simulink model "P_HIL_Virtual_Env"  (R2019b)
settings: Solver=VariableStepAuto  StartTime=0.0  StopTime=0.5  MaxStep=1e-6  RelTol=1e-3
undefined symbols (not defined in the file): Apd, Apd_i_dhs, Apd_u_dhs, C_dhs, f_sw, f_sw_dhs, In, L, L_dhs, L_drom, T_sw_dhs, Tid, Tid_i_dhs, Tid_u_dhs, U_DC
libraries: coordinate_transformations x19, simulink x6, PE_components x2
settings Model: SimulationMode=accelerator  Creator=kissd  LastModifiedBy=kissd

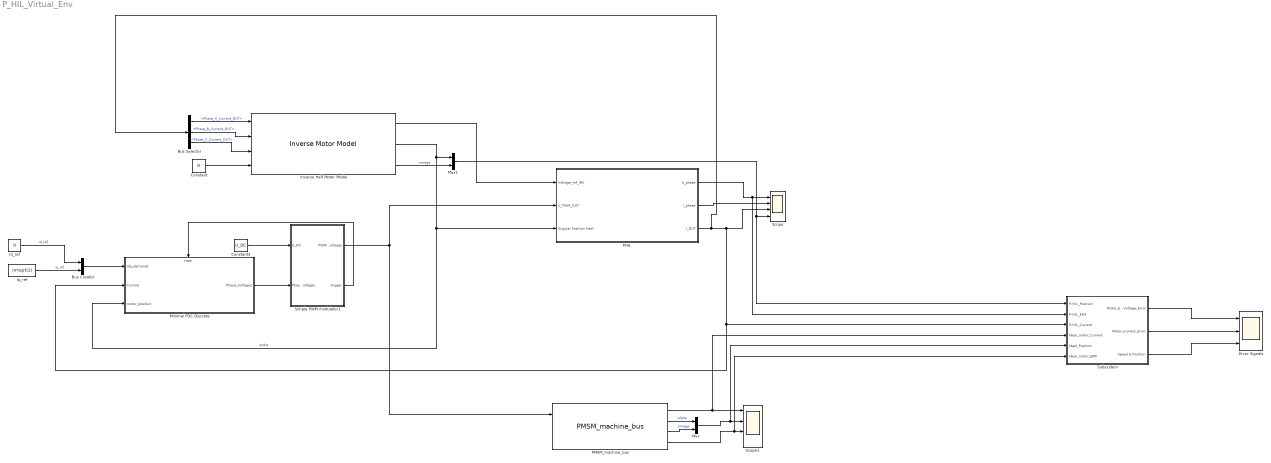
== system P_HIL_Virtual_Env ==
  Bus Creator : BusCreator  Inputs=2
  Bus Selector : BusSelector  OutputSignals=Phase_A_Current_DUT,Phase_B_Current_DUT,Phase_C_Current_DUT
  Constant : Constant  Value=0
  Constant3 : Constant  Value=U_DC
  Error Signals : Scope  NumInputPorts=3
  Inverse Half Motor Model : PE_components/Inverse Motor Model  SystemSampleTime=-1  Latency=0  AutoFrameSizeCalculation=off
  Minimal FOC Discrete : Subsystem  AncestorBlock=controllers/Minimal FOC Discrete
  Mux : Mux  Inputs=2
  Mux1 : Mux  Inputs=2
  PHIL : Subsystem
  PMSM_machine_bus : PE_components/PMSM_machine_bus  SystemSampleTime=-1  Latency=0  AutoFrameSizeCalculation=off
      link override Gain: Gain=1/Ld
      link override Gain3: Gain=1/Lq
      link override Gain8: Gain=Lq
  Scope : Scope  NumInputPorts=4
  Scope1 : Scope  NumInputPorts=4
  Simple PWM modulator1 : Subsystem  AncestorBlock=controllers/Simple PWM modulator
  Subsystem : Subsystem
  id_ref : Constant  Value=0
  iq_ref : Constant  Value=In*sqrt(2)
  wires:
  Constant3/1 -> Simple PWM modulator1/1(U_DC)
  id_ref/1 -> Bus Creator/1  "id_ref"
  iq_ref/1 -> Bus Creator/2  "iq_ref"
  Minimal FOC Discrete/1(Phase_Voltages) -> Simple PWM modulator1/2(Phase_Voltages)
  Simple PWM modulator1/2(trigger) -> Minimal FOC Discrete/Trigger
  Bus Creator/1 -> Minimal FOC Discrete/1(Idq_demands)
  Simple PWM modulator1/1(PWM_Voltages) -> PHIL/2("U_PWM_DUT "), PMSM_machine_bus/1
  PHIL/1(U_phase) -> Subsystem/2(P-HIL_EMF), Scope/1
  PHIL/2(I_phase) -> Scope/2
  PHIL/3(I_DUT) -> Bus Selector/1, Minimal FOC Discrete/2(Current), Subsystem/3(P-HIL_Current), Scope/3
  Inverse Half Motor Model/1 -> PHIL/1(Voltage_ref_INV)
  Bus Selector/1 -> Inverse Half Motor Model/1  "<Phase_A_Current_DUT>"
  Bus Selector/2 -> Inverse Half Motor Model/2  "<Phase_B_Current_DUT>"
  Bus Selector/3 -> Inverse Half Motor Model/3  "<Phase_C_Current_DUT>"
  Inverse Half Motor Model/3 -> Mux1/2  "omega"
  PMSM_machine_bus/1 -> Subsystem/4(Ideal_motor_Current), Scope1/1
  PMSM_machine_bus/4 -> Subsystem/6(Ideal_motor_EMF), Scope1/3
  PMSM_machine_bus/2 -> Mux/1  "alpha"
  PMSM_machine_bus/3 -> Mux/2  "omega"
  Mux/1 -> Subsystem/5(Ideal_Position), Scope1/2
  Inverse Half Motor Model/2 -> Mux1/1, Minimal FOC Discrete/3(motor_position), PHIL/3(Angular Position (rad))  "alpha"
  Mux1/1 -> Subsystem/1(P-HIL_Position), Scope/4
  Constant/1 -> Inverse Half Motor Model/4
  Subsystem/1(Motor_EMF_Voltage_Error) -> Error Signals/1
  Subsystem/2(Motor_Current_Error) -> Error Signals/2
  Subsystem/3(Speed & Position) -> Error Signals/3

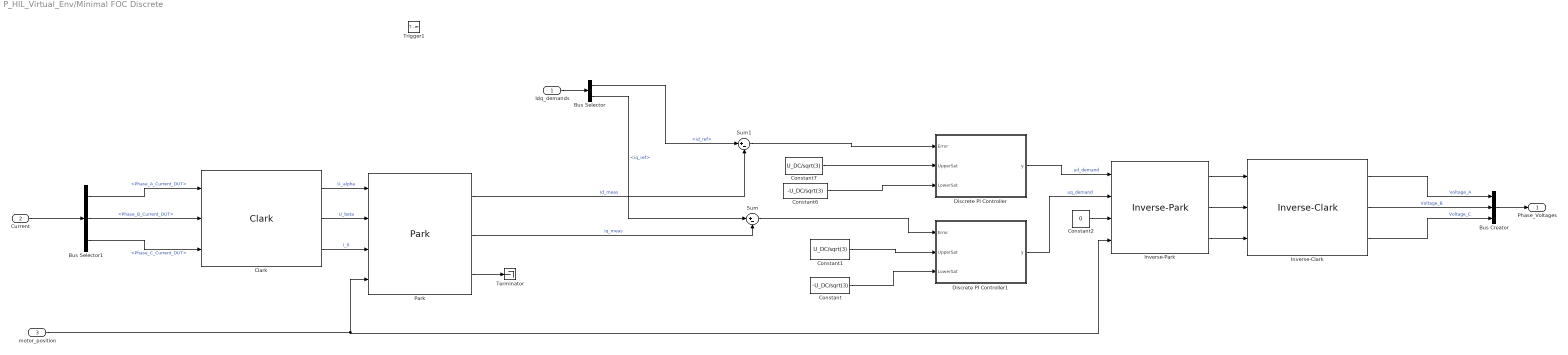
== system P_HIL_Virtual_Env/Minimal FOC Discrete ==
  Idq_demands : Inport
  Current : Inport  Port=2
  motor_position : Inport  Port=3
  Trigger1 : TriggerPort  TriggerType=either  VariantControl=Variant  PortDimensions=1
  Bus Creator : BusCreator  Inputs=3
  Bus Selector : BusSelector  OutputSignals=id_ref,iq_ref
  Bus Selector1 : BusSelector  OutputSignals=Phase_A_Current_DUT,Phase_B_Current_DUT,Phase_C_Current_DUT
  Clark : coordinate_transformations/Clark  SystemSampleTime=-1  Latency=0  AutoFrameSizeCalculation=off
  Constant : Constant  Value=-U_DC/sqrt(3)
  Constant1 : Constant  Value=U_DC/sqrt(3)
  Constant2 : Constant  Value=0
  Constant6 : Constant  Value=-U_DC/sqrt(3)
  Constant7 : Constant  Value=U_DC/sqrt(3)
  Discrete PI Controller : Subsystem  AncestorBlock=controllers/Discrete PI Controller  mask(Continous PI Controller){Apd=Apd, Tid=Tid, fs=f_sw}
      mask prompts: Apd "Proprotional Gain"; Tid "Integration Time"; fs "fsw"
      mask help: Continous PI Controller description.
  Discrete PI Controller1 : Subsystem  AncestorBlock=controllers/Discrete PI Controller  mask(Continous PI Controller){Apd=Apd, Tid=Tid, fs=f_sw}
      mask prompts: Apd "Proprotional Gain"; Tid "Integration Time"; fs "fsw"
      mask help: Continous PI Controller description.
  Inverse-Clark : coordinate_transformations/Inverse-Clark  SystemSampleTime=-1  Latency=0  AutoFrameSizeCalculation=off
  Inverse-Park : coordinate_transformations/Inverse-Park  SystemSampleTime=-1  Latency=0  AutoFrameSizeCalculation=off
  Park : coordinate_transformations/Park  SystemSampleTime=-1  Latency=0  AutoFrameSizeCalculation=off
  Sum : Sum  Inputs=|+-
  Sum1 : Sum  Inputs=|+-
  Terminator : Terminator
  Phase_Voltages : Outport
  wires:
  Discrete PI Controller1/1(y) -> Inverse-Park/2  "uq_demand"
  Inverse-Park/2 -> Inverse-Clark/2
  Inverse-Park/3 -> Inverse-Clark/3
  Park/2 -> Sum/2  "Iq_meas"
  Constant7/1 -> Discrete PI Controller/2(UpperSat)
  Clark/1 -> Park/1  "U_alpha"
  Inverse-Clark/3 -> Bus Creator/3  "Voltage_C"
  Constant1/1 -> Discrete PI Controller1/2(UpperSat)
  Sum/1 -> Discrete PI Controller1/1(Error)
  Inverse-Park/1 -> Inverse-Clark/1
  Constant6/1 -> Discrete PI Controller/3(LowerSat)
  motor_position/1 -> Park/4, Inverse-Park/4
  Park/1 -> Sum1/2  "Id_meas"
  Discrete PI Controller/1(y) -> Inverse-Park/1  "ud_demand"
  Constant/1 -> Discrete PI Controller1/3(LowerSat)
  Sum1/1 -> Discrete PI Controller/1(Error)
  Clark/2 -> Park/2  "U_beta"
  Bus Selector/2 -> Sum/1  "<iq_ref>"
  Clark/3 -> Park/3  "I_0"
  Park/3 -> Terminator/1
  Inverse-Clark/2 -> Bus Creator/2  "Voltage_B"
  Bus Selector/1 -> Sum1/1  "<id_ref>"
  Inverse-Clark/1 -> Bus Creator/1  "Voltage_A"
  Current/1 -> Bus Selector1/1
  Constant2/1 -> Inverse-Park/3
  Idq_demands/1 -> Bus Selector/1
  Bus Creator/1 -> Phase_Voltages/1
  Bus Selector1/2 -> Clark/2  "<Phase_B_Current_DUT>"
  Bus Selector1/1 -> Clark/1  "<Phase_A_Current_DUT>"
  Bus Selector1/3 -> Clark/3  "<Phase_C_Current_DUT>"

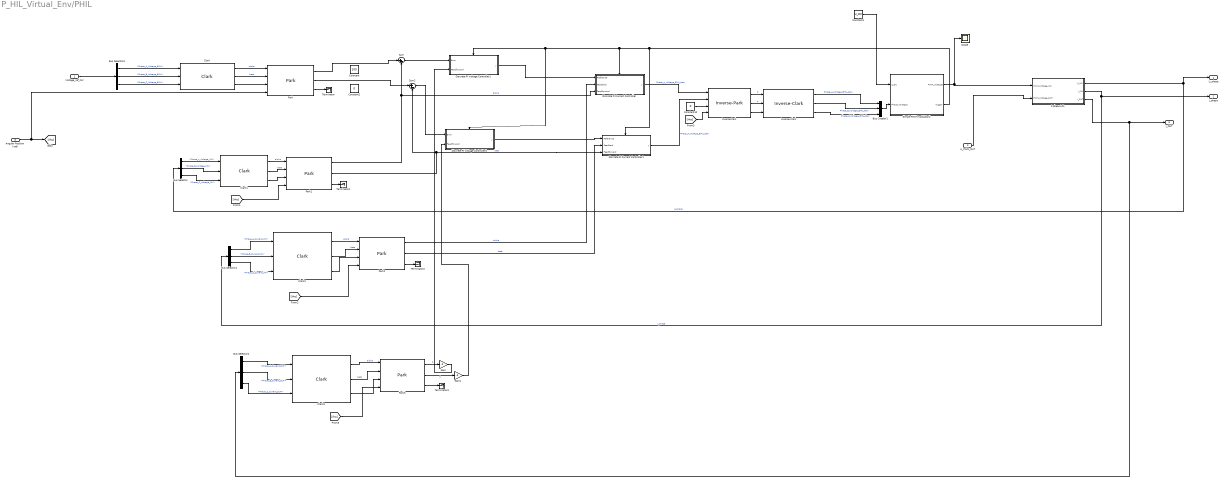
== system P_HIL_Virtual_Env/PHIL ==
  Voltage_ref_INV : Inport
  "U_PWM_DUT " : Inport  Port=2
  Angular Position (rad) : Inport  Port=3
  3 phase LCL : Subsystem
  Bus Creator1 : BusCreator  Inputs=3
  Bus Selector : BusSelector  OutputSignals=Phase_A_Voltage_INV,Phase_B_Voltage_INV,Phase_C_Voltage_INV
  Bus Selector1 : BusSelector  OutputSignals=Phase_A_Current_INV,Phase_B_Current_INV,Phase_C_Current_INV
  Bus Selector2 : BusSelector  OutputSignals=Phase_A_Current_DUT,Phase_B_Current_DUT,Phase_C_Current_DUT
  Bus Selector3 : BusSelector  OutputSignals=Phase_A_Voltage_EMU,Phase_B_Voltage_EMU,Phase_C_Voltage_EMU
  Clark{,1..3} (4 alike) : coordinate_transformations/Clark  SystemSampleTime=-1  Latency=0  AutoFrameSizeCalculation=off
  Constant : Constant  Value=100
  Constant1 : Constant  Value=U_DC
  Constant10 : Constant  Value=0
  Constant2 : Constant  Value=0
  Discrete PI Current Controller : Subsystem  AncestorBlock=controllers/Discrete PI Controller  mask(Continous PI Controller){Apd=Apd_i_dhs, Tid=Tid_i_dhs, fs=f_sw_dhs, UpperSat=U_DC, LowerSat=-U_DC}
      mask prompts: Apd "Proprotional Gain"; Tid "Integration Time"; fs "fsw"; UpperSat "Max. Saturation"; LowerSat "Min. Saturation"
      mask help: Continous PI Controller description.
  Discrete PI Current Controller1 : Subsystem  AncestorBlock=controllers/Discrete PI Controller  mask(Continous PI Controller){Apd=Apd_i_dhs, Tid=Tid_i_dhs, fs=f_sw_dhs, UpperSat=U_DC, LowerSat=-U_DC}
      mask prompts: Apd "Proprotional Gain"; Tid "Integration Time"; fs "fsw"; UpperSat "Max. Saturation"; LowerSat "Min. Saturation"
      mask help: Continous PI Controller description.
  Discrete PI Voltage Controller1 : Subsystem  AncestorBlock=controllers/Discrete PI Controller  mask(Continous PI Controller){Apd=Apd_u_dhs, Tid=Tid_u_dhs, fs=f_sw_dhs, UpperSat=300, LowerSat=-300}
      mask prompts: Apd "Proprotional Gain"; Tid "Integration Time"; fs "fsw"; UpperSat "Max. Saturation"; LowerSat "Min. Saturation"
      mask help: Continous PI Controller description.
  Discrete PI Voltage Controller3 : Subsystem  AncestorBlock=controllers/Discrete PI Controller  mask(Continous PI Controller){Apd=Apd_u_dhs, Tid=Tid_u_dhs, fs=f_sw_dhs, UpperSat=300, LowerSat=-300}
      mask prompts: Apd "Proprotional Gain"; Tid "Integration Time"; fs "fsw"; UpperSat "Max. Saturation"; LowerSat "Min. Saturation"
      mask help: Continous PI Controller description.
  Gain : Gain  Gain=-1
  Gain1 : Gain  Gain=-1
  Inverse-Clark : coordinate_transformations/Inverse-Clark  SystemSampleTime=-1  Latency=0  AutoFrameSizeCalculation=off
  Inverse-Park : coordinate_transformations/Inverse-Park  SystemSampleTime=-1  Latency=0  AutoFrameSizeCalculation=off
  Park{,1..3} (4 alike) : coordinate_transformations/Park  SystemSampleTime=-1  Latency=0  AutoFrameSizeCalculation=off
  Scope : Scope
  Simple PWM modulator2 : Subsystem  AncestorBlock=controllers/Simple PWM modulator
  Sum : Sum  Inputs=|+-
  Sum2 : Sum  Inputs=|+-
  Terminator{,1..3} (4 alike) : Terminator
  U_phase : Outport
  I_phase : Outport  Port=2
  I_DUT : Outport  Port=3
  wires:
  Sum2/1 -> Discrete PI Voltage Controller3/1(Error)
  Inverse-Clark/1 -> Bus Creator1/1  "Phase_A_Voltage_EMU_dem"
  Inverse-Park/2 -> Inverse-Clark/2  "q"
  3 phase LCL/1(U_INV) -> Bus Selector/1, U_phase/1  "U_phase"
  3 phase LCL/3(I_DUT) -> Bus Selector2/1, I_DUT/1
  Simple PWM modulator2/1(PWM_Voltages) -> Scope/1, 3 phase LCL/1(PWM_Voltage_INV)
  "U_PWM_DUT "/1 -> 3 phase LCL/2(PWM_Voltage_DUT)
  Park1/1 -> Discrete PI Current Controller/3(Feedforward), Sum/2  "alpha"
  [rho] -> Inverse-Park/4
  Constant10/1 -> Inverse-Park/3
  Clark2/1 -> Park2/1  "alpha"
  Discrete PI Current Controller1/1(y) -> Inverse-Park/2  "Phase_A_Voltage_EMU_dem"
  Discrete PI Current Controller/1(y) -> Inverse-Park/1  "Phase_A_Voltage_EMU_dem"
  Constant1/1 -> Simple PWM modulator2/1(U_DC)
  Simple PWM modulator2/2(trigger) -> Discrete PI Current Controller1/Trigger, Discrete PI Current Controller/Trigger, Discrete PI Voltage Controller1/Trigger, Discrete PI Voltage Controller3/Trigger
  Park1/2 -> Discrete PI Current Controller1/3(Feedforward), Sum2/2  "beta"
  Clark3/2 -> Park3/2  "beta"
  Inverse-Clark/2 -> Bus Creator1/2  "Phase_B_Voltage_EMU_dem"
  Park1/3 -> Terminator1/1
  Clark1/1 -> Park1/1  "alpha"
  Bus Selector1/3 -> Clark2/3  "<Phase_C_Current_INV>"
  Park2/3 -> Terminator2/1
  Clark1/3 -> Park1/3
  Park2/2 -> Discrete PI Current Controller1/2(Feedback)  "beta"
  Sum/1 -> Discrete PI Voltage Controller1/1(Error)
  Clark1/2 -> Park1/2  "beta"
  Clark3/1 -> Park3/1  "alpha"
  3 phase LCL/2(I_INV) -> I_phase/1, Bus Selector1/1  "I_phase"
  Park2/1 -> Discrete PI Current Controller/2(Feedback)  "alpha"
  Clark3/3 -> Park3/3
  Voltage_ref_INV/1 -> Bus Selector3/1
  Clark2/2 -> Park2/2  "beta"
  Discrete PI Voltage Controller3/1(y) -> Discrete PI Current Controller1/1(Reference)
  Inverse-Clark/3 -> Bus Creator1/3  "Phase_C_Voltage_EMU_dem"
  Clark/1 -> Park/1  "alpha"
  Bus Creator1/1 -> Simple PWM modulator2/2(Phase_Voltages)
  Bus Selector1/1 -> Clark2/1  "<Phase_A_Current_INV>"
  Inverse-Park/1 -> Inverse-Clark/1  "d"
  Bus Selector/3 -> Clark1/3  "<Phase_C_Voltage_INV>"
  Bus Selector/1 -> Clark1/1  "<Phase_A_Voltage_INV>"
  Bus Selector/2 -> Clark1/2  "<Phase_B_Voltage_INV>"
  Park3/3 -> Terminator3/1
  Discrete PI Voltage Controller1/1(y) -> Discrete PI Current Controller/1(Reference)
  Clark2/3 -> Park2/3
  Bus Selector1/2 -> Clark2/2  "<Phase_B_Current_INV>"
  Clark/3 -> Park/3
  Inverse-Park/3 -> Inverse-Clark/3
  Park/3 -> Terminator/1
  Clark/2 -> Park/2  "beta"
  Bus Selector3/1 -> Clark/1  "<Phase_A_Voltage_EMU>"
  Bus Selector3/2 -> Clark/2  "<Phase_B_Voltage_EMU>"
  Bus Selector3/3 -> Clark/3  "<Phase_C_Voltage_EMU>"
  Angular Position (rad)/1 -> Park/4, [rho]
  [rho] -> Park1/4
  [rho] -> Park2/4
  [rho] -> Park3/4
  Park/1 -> Sum/1
  Park/2 -> Sum2/1
  Bus Selector2/1 -> Clark3/1  "<Phase_A_Current_DUT>"
  Bus Selector2/2 -> Clark3/2  "<Phase_B_Current_DUT>"
  Bus Selector2/3 -> Clark3/3  "<Phase_C_Current_DUT>"
  Park3/1 -> Gain/1  "d"
  Park3/2 -> Gain1/1  "q"
  Gain/1 -> Discrete PI Voltage Controller1/2(Feedforward)
  Gain1/1 -> Discrete PI Voltage Controller3/2(Feedforward)

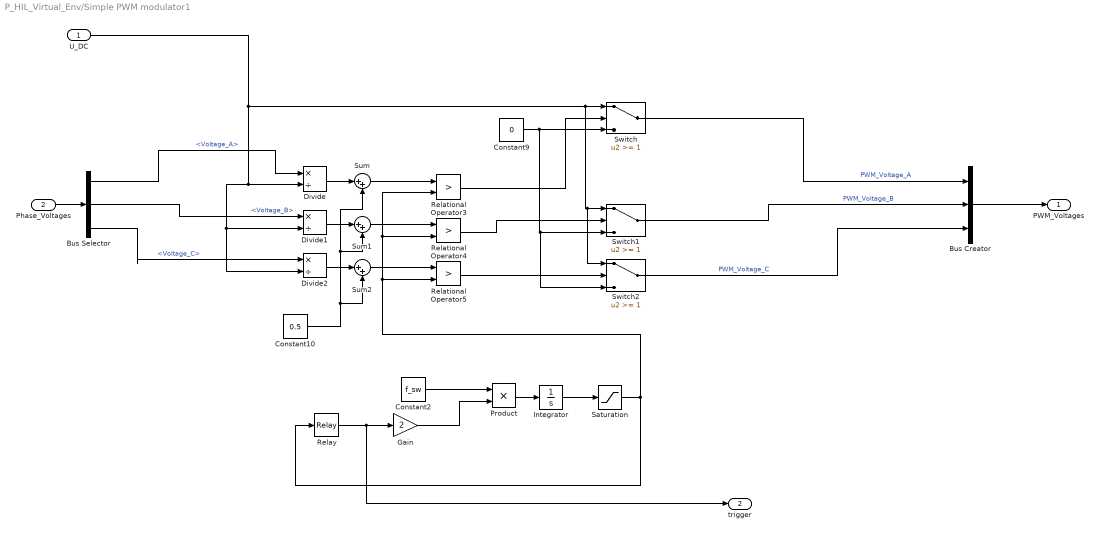
== system P_HIL_Virtual_Env/Simple PWM modulator1 ==
  U_DC : Inport
  Phase_Voltages : Inport  Port=2
  Bus Creator : BusCreator  Inputs=3
  Bus Selector : BusSelector  OutputSignals=Voltage_A,Voltage_B,Voltage_C
  Constant10 : Constant  Value=0.5
  Constant2 : Constant  Value=f_sw
  Constant9 : Constant  Value=0
  Divide : Product  Inputs=*/
  Divide1 : Product  Inputs=*/
  Divide2 : Product  Inputs=*/
  Gain : Gain  Gain=2
  Integrator : Integrator
  Product : Product
  Relational Operator3 : RelationalOperator  Operator=>  OutDataTypeStr=boolean  RndMeth=Simplest
  Relational Operator4 : RelationalOperator  Operator=>  OutDataTypeStr=boolean  RndMeth=Simplest
  Relational Operator5 : RelationalOperator  Operator=>  OutDataTypeStr=boolean  RndMeth=Simplest
  Relay : Relay  OnSwitchValue=1  OffSwitchValue=0  OnOutputValue=-1  OffOutputValue=1
  Saturation : Saturate  UpperLimit=1  LowerLimit=0
  Sum : Sum  Inputs=|++
  Sum1 : Sum  Inputs=|++
  Sum2 : Sum  Inputs=|++
  Switch : Switch  Threshold=1
  Switch1 : Switch  Threshold=1
  Switch2 : Switch  Threshold=1
  PWM_Voltages : Outport
  trigger : Outport  Port=2
  wires:
  Constant2/1 -> Product/1
  Sum1/1 -> Relational Operator4/1
  Product/1 -> Integrator/1
  Relational Operator5/1 -> Switch2/2
  Integrator/1 -> Saturation/1
  Divide1/1 -> Sum1/1
  Saturation/1 -> Relational Operator3/2, Relational Operator4/2, Relational Operator5/2, Relay/1
  Relay/1 -> trigger/1, Gain/1
  Constant10/1 -> Sum2/2, Sum1/2, Sum/2
  Relational Operator3/1 -> Switch/2
  Switch/1 -> Bus Creator/1  "PWM_Voltage_A"
  Bus Selector/2 -> Divide1/1  "<Voltage_B>"
  Switch2/1 -> Bus Creator/3  "PWM_Voltage_C"
  Constant9/1 -> Switch2/3, Switch1/3, Switch/3
  Relational Operator4/1 -> Switch1/2
  Gain/1 -> Product/2
  Sum/1 -> Relational Operator3/1
  Divide2/1 -> Sum2/1
  Divide/1 -> Sum/1
  Sum2/1 -> Relational Operator5/1
  Bus Selector/3 -> Divide2/1  "<Voltage_C>"
  Bus Selector/1 -> Divide/1  "<Voltage_A>"
  Switch1/1 -> Bus Creator/2  "PWM_Voltage_B"
  U_DC/1 -> Switch2/1, Switch1/1, Switch/1, Divide2/2, Divide1/2, Divide/2
  Phase_Voltages/1 -> Bus Selector/1
  Bus Creator/1 -> PWM_Voltages/1

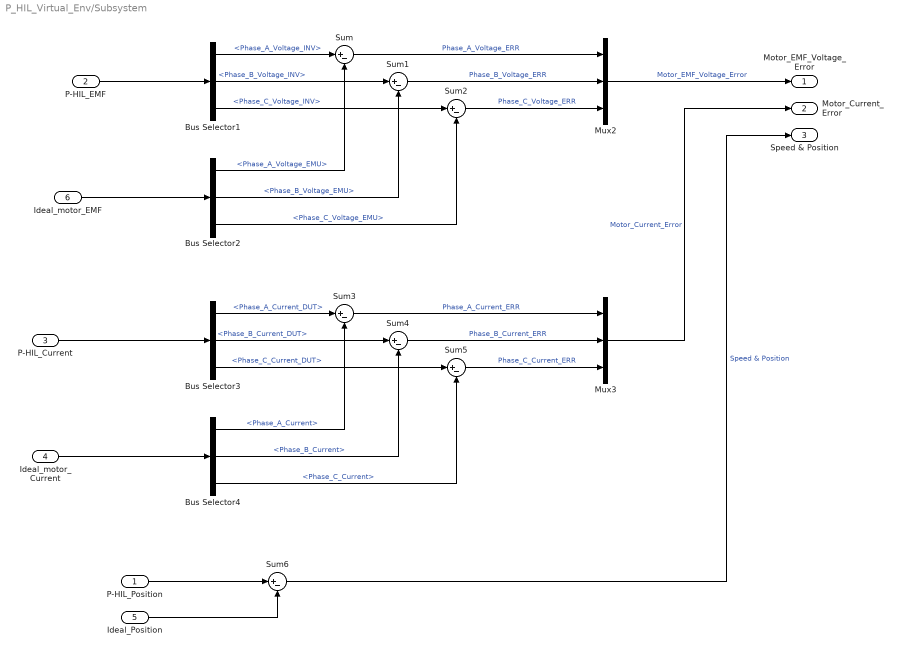
== system P_HIL_Virtual_Env/Subsystem ==
  P-HIL_Position : Inport
  P-HIL_EMF : Inport  Port=2
  P-HIL_Current : Inport  Port=3
  Ideal_motor_Current : Inport  Port=4
  Ideal_Position : Inport  Port=5
  Ideal_motor_EMF : Inport  Port=6
  Bus Selector1 : BusSelector  OutputSignals=Phase_A_Voltage_INV,Phase_B_Voltage_INV,Phase_C_Voltage_INV
  Bus Selector2 : BusSelector  OutputSignals=Phase_A_Voltage_EMU,Phase_B_Voltage_EMU,Phase_C_Voltage_EMU
  Bus Selector3 : BusSelector  OutputSignals=Phase_A_Current_DUT,Phase_B_Current_DUT,Phase_C_Current_DUT
  Bus Selector4 : BusSelector  OutputSignals=Phase_A_Current,Phase_B_Current,Phase_C_Current
  Mux2 : Mux  Inputs=3
  Mux3 : Mux  Inputs=3
  Sum{,1..6} (7 alike) : Sum  Inputs=|+-
  Motor_EMF_Voltage_Error : Outport
  Motor_Current_Error : Outport  Port=2
  Speed & Position : Outport  Port=3
  wires:
  P-HIL_Position/1 -> Sum6/1
  Sum1/1 -> Mux2/2  "Phase_B_Voltage_ERR"
  Sum2/1 -> Mux2/3  "Phase_C_Voltage_ERR"
  Ideal_Position/1 -> Sum6/2
  Bus Selector3/1 -> Sum3/1  "<Phase_A_Current_DUT>"
  Bus Selector1/1 -> Sum/1  "<Phase_A_Voltage_INV>"
  Sum/1 -> Mux2/1  "Phase_A_Voltage_ERR"
  Bus Selector2/3 -> Sum2/2  "<Phase_C_Voltage_EMU>"
  Bus Selector1/3 -> Sum2/1  "<Phase_C_Voltage_INV>"
  Bus Selector3/2 -> Sum4/1  "<Phase_B_Current_DUT>"
  Ideal_motor_EMF/1 -> Bus Selector2/1
  Bus Selector1/2 -> Sum1/1  "<Phase_B_Voltage_INV>"
  Sum5/1 -> Mux3/3  "Phase_C_Current_ERR"
  Bus Selector4/1 -> Sum3/2  "<Phase_A_Current>"
  Sum4/1 -> Mux3/2  "Phase_B_Current_ERR"
  Sum3/1 -> Mux3/1  "Phase_A_Current_ERR"
  Bus Selector4/3 -> Sum5/2  "<Phase_C_Current>"
  Bus Selector4/2 -> Sum4/2  "<Phase_B_Current>"
  Bus Selector2/1 -> Sum/2  "<Phase_A_Voltage_EMU>"
  Bus Selector3/3 -> Sum5/1  "<Phase_C_Current_DUT>"
  Bus Selector2/2 -> Sum1/2  "<Phase_B_Voltage_EMU>"
  Sum6/1 -> Speed & Position/1  "Speed & Position"
  Ideal_motor_Current/1 -> Bus Selector4/1
  Mux3/1 -> Motor_Current_Error/1  "Motor_Current_Error"
  P-HIL_Current/1 -> Bus Selector3/1
  P-HIL_EMF/1 -> Bus Selector1/1
  Mux2/1 -> Motor_EMF_Voltage_Error/1  "Motor_EMF_Voltage_Error"

== system P_HIL_Virtual_Env/Minimal FOC Discrete/Discrete PI Controller ==
  Error : Inport
  UpperSat : Inport  Port=2
  LowerSat : Inport  Port=3
  Delay : Delay  DelayLength=1
  Delay1 : Delay  DelayLength=1
  Delay2 : Delay  DelayLength=1
  Gain1 : Gain  Gain=Apd
  Gain2 : Gain  Gain=1/(2*fs*Tid)
  Saturation Dynamic : simulink/Discontinuities/Saturation Dynamic  OutMin=[]  OutMax=[]  OutDataTypeStr=Inherit: Same as second input  OutDataType=fixdt(1, 16)  OutScaling=2^-10  DoSatur=off
  Sum : Sum  Inputs=|-+
  Sum1 : Sum  Inputs=+++
  y : Outport
  wires:
  Delay2/1 -> y/1
  Delay1/1 -> Sum1/1
  Gain2/1 -> Sum1/3
  Sum/1 -> Sum1/2
  Delay/1 -> Sum/1
  LowerSat/1 -> Saturation Dynamic/3
  UpperSat/1 -> Saturation Dynamic/1
  Saturation Dynamic/1 -> Delay2/1, Delay1/1
  Sum1/1 -> Saturation Dynamic/2
  Gain1/1 -> Delay/1, Sum/2, Gain2/1
  Error/1 -> Gain1/1

== system P_HIL_Virtual_Env/Minimal FOC Discrete/Discrete PI Controller1 ==
  Error : Inport
  UpperSat : Inport  Port=2
  LowerSat : Inport  Port=3
  Delay : Delay  DelayLength=1
  Delay1 : Delay  DelayLength=1
  Delay2 : Delay  DelayLength=1
  Gain1 : Gain  Gain=Apd
  Gain2 : Gain  Gain=1/(2*fs*Tid)
  Saturation Dynamic : simulink/Discontinuities/Saturation Dynamic  OutMin=[]  OutMax=[]  OutDataTypeStr=Inherit: Same as second input  OutDataType=fixdt(1, 16)  OutScaling=2^-10  DoSatur=off
  Sum : Sum  Inputs=|-+
  Sum1 : Sum  Inputs=+++
  y : Outport
  wires:
  Delay2/1 -> y/1
  Delay1/1 -> Sum1/1
  Gain2/1 -> Sum1/3
  Sum/1 -> Sum1/2
  Delay/1 -> Sum/1
  LowerSat/1 -> Saturation Dynamic/3
  UpperSat/1 -> Saturation Dynamic/1
  Saturation Dynamic/1 -> Delay2/1, Delay1/1
  Sum1/1 -> Saturation Dynamic/2
  Gain1/1 -> Delay/1, Sum/2, Gain2/1
  Error/1 -> Gain1/1

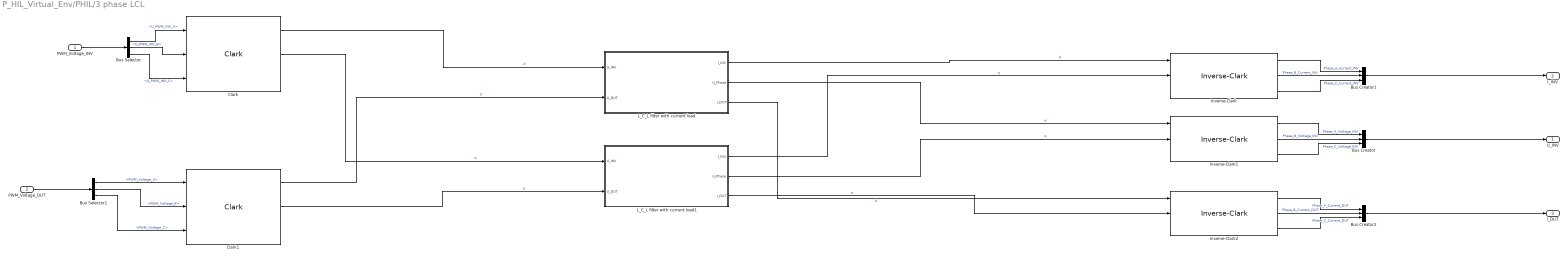
== system P_HIL_Virtual_Env/PHIL/3 phase LCL ==
  PWM_Voltage_INV : Inport
  PWM_Voltage_DUT : Inport  Port=2
  Bus Creator : BusCreator  Inputs=3
  Bus Creator1 : BusCreator  Inputs=3
  Bus Creator2 : BusCreator  Inputs=3
  Bus Selector : BusSelector  OutputSignals=U_PWM_INV_A,U_PWM_INV_B,U_PWM_INV_C
  Bus Selector1 : BusSelector  OutputSignals=PWM_Voltage_A,PWM_Voltage_B,PWM_Voltage_C
  Clark : coordinate_transformations/Clark  SystemSampleTime=-1  Latency=0  AutoFrameSizeCalculation=off
  Clark1 : coordinate_transformations/Clark  SystemSampleTime=-1  Latency=0  AutoFrameSizeCalculation=off
  Inverse-Clark : coordinate_transformations/Inverse-Clark  SystemSampleTime=-1  Latency=0  AutoFrameSizeCalculation=off
  Inverse-Clark1 : coordinate_transformations/Inverse-Clark  SystemSampleTime=-1  Latency=0  AutoFrameSizeCalculation=off
  Inverse-Clark2 : coordinate_transformations/Inverse-Clark  SystemSampleTime=-1  Latency=0  AutoFrameSizeCalculation=off
  L_C_L filter with current load : Subsystem
  L_C_L filter with current load1 : Subsystem
  U_INV : Outport
  I_INV : Outport  Port=2
  I_DUT : Outport  Port=3
  wires:
  PWM_Voltage_INV/1 -> Bus Selector/1
  Bus Creator/1 -> U_INV/1
  Bus Creator1/1 -> I_INV/1
  PWM_Voltage_DUT/1 -> Bus Selector1/1
  Bus Selector/2 -> Clark/2  "<U_PWM_INV_B>"
  Bus Selector/1 -> Clark/1  "<U_PWM_INV_A>"
  Bus Selector/3 -> Clark/3  "<U_PWM_INV_C>"
  Inverse-Clark1/2 -> Bus Creator/2  "Phase_B_Voltage_INV"
  Inverse-Clark1/1 -> Bus Creator/1  "Phase_A_Voltage_INV"
  Inverse-Clark1/3 -> Bus Creator/3  "Phase_C_Voltage_INV"
  Inverse-Clark/2 -> Bus Creator1/2  "Phase_B_Current_INV"
  Inverse-Clark/1 -> Bus Creator1/1  "Phase_A_Current_INV"
  Inverse-Clark/3 -> Bus Creator1/3  "Phase_C_Current_INV"
  Inverse-Clark2/1 -> Bus Creator2/1  "Phase_A_Current_DUT"
  Inverse-Clark2/2 -> Bus Creator2/2  "Phase_B_Current_DUT"
  Inverse-Clark2/3 -> Bus Creator2/3  "Phase_C_Current_DUT"
  Bus Creator2/1 -> I_DUT/1
  Bus Selector1/1 -> Clark1/1  "<PWM_Voltage_A>"
  Bus Selector1/2 -> Clark1/2  "<PWM_Voltage_B>"
  Bus Selector1/3 -> Clark1/3  "<PWM_Voltage_C>"
  Clark/1 -> L_C_L filter with current load/1(U_INV)  "d"
  Clark/2 -> L_C_L filter with current load1/1(U_INV)  "q"
  Clark1/1 -> L_C_L filter with current load/2(U_DUT)  "d"
  Clark1/2 -> L_C_L filter with current load1/2(U_DUT)  "q"
  L_C_L filter with current load/1(I_INV) -> Inverse-Clark/1  "d"
  L_C_L filter with current load1/1(I_INV) -> Inverse-Clark/2  "q"
  L_C_L filter with current load/2(U_Phase) -> Inverse-Clark1/1  "d"
  L_C_L filter with current load1/2(U_Phase) -> Inverse-Clark1/2  "q"
  L_C_L filter with current load/3(I_DUT) -> Inverse-Clark2/1  "d"
  L_C_L filter with current load1/3(I_DUT) -> Inverse-Clark2/2  "q"

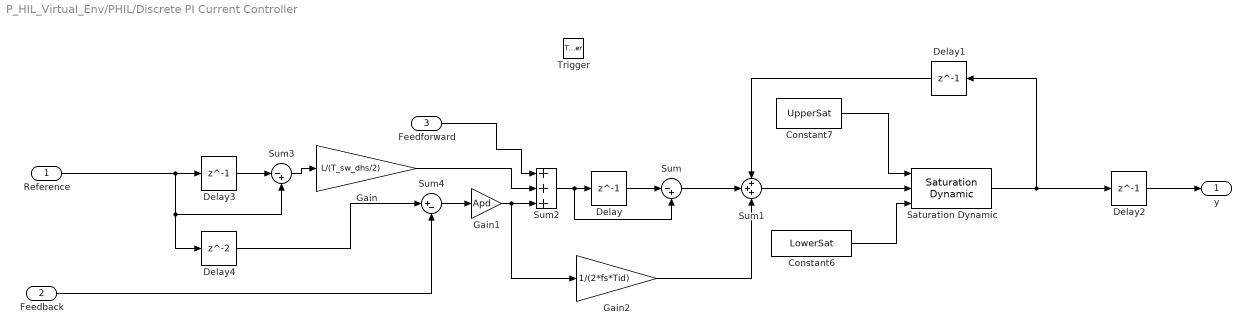
== system P_HIL_Virtual_Env/PHIL/Discrete PI Current Controller ==
  Reference : Inport
  Feedback : Inport  Port=2
  Feedforward : Inport  Port=3
  Trigger : TriggerPort  TriggerType=either  VariantControl=Variant  PortDimensions=1
  Constant6 : Constant  Value=LowerSat
  Constant7 : Constant  Value=UpperSat
  Delay{,1..3} (4 alike) : Delay  DelayLength=1
  Delay4 : Delay
  Gain : Gain  Gain=L/(T_sw_dhs/2)
  Gain1 : Gain  Gain=Apd
  Gain2 : Gain  Gain=1/(2*fs*Tid)
  Saturation Dynamic : simulink/Discontinuities/Saturation Dynamic  OutMin=[]  OutMax=[]  OutDataTypeStr=Inherit: Same as second input  OutDataType=fixdt(1, 16)  OutScaling=2^-10  DoSatur=off
  Sum : Sum  Inputs=|-+
  Sum1 : Sum  Inputs=+++
  Sum2 : Sum  Inputs=+++
  Sum3 : Sum  Inputs=|-+
  Sum4 : Sum  Inputs=|+-
  y : Outport
  wires:
  Gain1/1 -> Sum2/3, Gain2/1
  Sum1/1 -> Saturation Dynamic/2
  Saturation Dynamic/1 -> Delay1/1, Delay2/1
  Constant7/1 -> Saturation Dynamic/1
  Constant6/1 -> Saturation Dynamic/3
  Delay/1 -> Sum/1
  Sum/1 -> Sum1/2
  Gain2/1 -> Sum1/3
  Delay1/1 -> Sum1/1
  Delay2/1 -> y/1
  Sum2/1 -> Sum/2, Delay/1
  Feedforward/1 -> Sum2/1
  Delay3/1 -> Sum3/1
  Reference/1 -> Sum3/2, Delay4/1, Delay3/1
  Sum4/1 -> Gain1/1
  Sum3/1 -> Gain/1
  Gain/1 -> Sum2/2
  Feedback/1 -> Sum4/2
  Delay4/1 -> Sum4/1

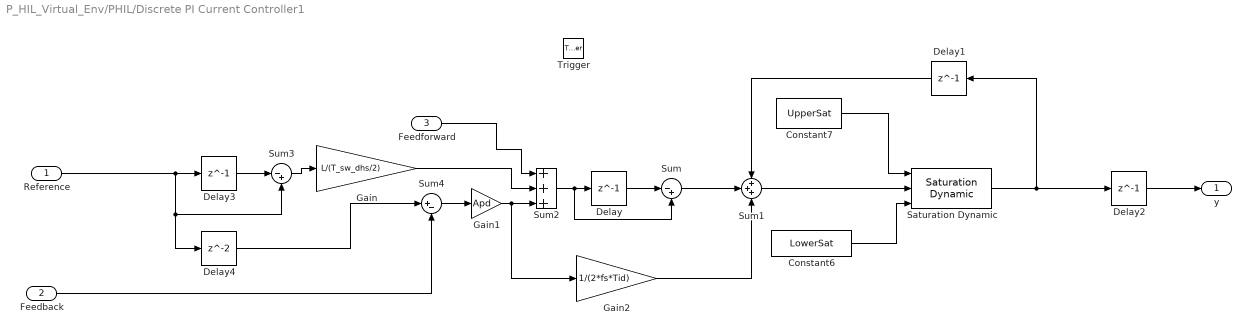
== system P_HIL_Virtual_Env/PHIL/Discrete PI Current Controller1 ==
  Reference : Inport
  Feedback : Inport  Port=2
  Feedforward : Inport  Port=3
  Trigger : TriggerPort  TriggerType=either  VariantControl=Variant  PortDimensions=1
  Constant6 : Constant  Value=LowerSat
  Constant7 : Constant  Value=UpperSat
  Delay{,1..3} (4 alike) : Delay  DelayLength=1
  Delay4 : Delay
  Gain : Gain  Gain=L/(T_sw_dhs/2)
  Gain1 : Gain  Gain=Apd
  Gain2 : Gain  Gain=1/(2*fs*Tid)
  Saturation Dynamic : simulink/Discontinuities/Saturation Dynamic  OutMin=[]  OutMax=[]  OutDataTypeStr=Inherit: Same as second input  OutDataType=fixdt(1, 16)  OutScaling=2^-10  DoSatur=off
  Sum : Sum  Inputs=|-+
  Sum1 : Sum  Inputs=+++
  Sum2 : Sum  Inputs=+++
  Sum3 : Sum  Inputs=|-+
  Sum4 : Sum  Inputs=|+-
  y : Outport
  wires:
  Gain1/1 -> Sum2/3, Gain2/1
  Sum1/1 -> Saturation Dynamic/2
  Saturation Dynamic/1 -> Delay1/1, Delay2/1
  Constant7/1 -> Saturation Dynamic/1
  Constant6/1 -> Saturation Dynamic/3
  Delay/1 -> Sum/1
  Sum/1 -> Sum1/2
  Gain2/1 -> Sum1/3
  Delay1/1 -> Sum1/1
  Delay2/1 -> y/1
  Sum2/1 -> Sum/2, Delay/1
  Feedforward/1 -> Sum2/1
  Delay3/1 -> Sum3/1
  Reference/1 -> Sum3/2, Delay4/1, Delay3/1
  Sum4/1 -> Gain1/1
  Sum3/1 -> Gain/1
  Gain/1 -> Sum2/2
  Feedback/1 -> Sum4/2
  Delay4/1 -> Sum4/1

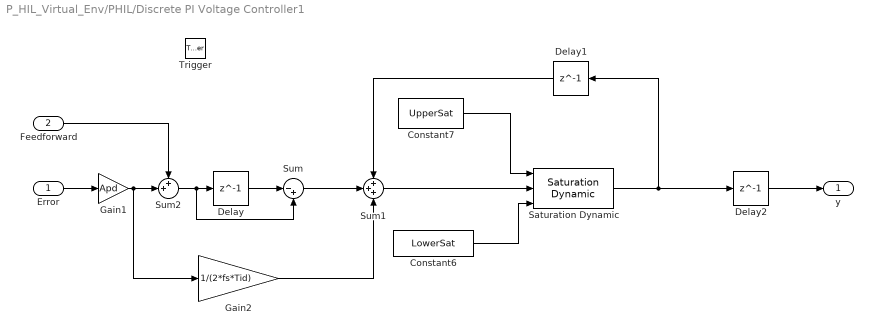
== system P_HIL_Virtual_Env/PHIL/Discrete PI Voltage Controller1 ==
  Error : Inport
  Feedforward : Inport  Port=2
  Trigger : TriggerPort  TriggerType=either  VariantControl=Variant  PortDimensions=1
  Constant6 : Constant  Value=LowerSat
  Constant7 : Constant  Value=UpperSat
  Delay : Delay  DelayLength=1
  Delay1 : Delay  DelayLength=1
  Delay2 : Delay  DelayLength=1
  Gain1 : Gain  Gain=Apd
  Gain2 : Gain  Gain=1/(2*fs*Tid)
  Saturation Dynamic : simulink/Discontinuities/Saturation Dynamic  OutMin=[]  OutMax=[]  OutDataTypeStr=Inherit: Same as second input  OutDataType=fixdt(1, 16)  OutScaling=2^-10  DoSatur=off
  Sum : Sum  Inputs=|-+
  Sum1 : Sum  Inputs=+++
  Sum2 : Sum  Inputs=++|
  y : Outport
  wires:
  Error/1 -> Gain1/1
  Gain1/1 -> Sum2/2, Gain2/1
  Sum1/1 -> Saturation Dynamic/2
  Saturation Dynamic/1 -> Delay1/1, Delay2/1
  Constant7/1 -> Saturation Dynamic/1
  Constant6/1 -> Saturation Dynamic/3
  Delay/1 -> Sum/1
  Sum/1 -> Sum1/2
  Gain2/1 -> Sum1/3
  Delay1/1 -> Sum1/1
  Delay2/1 -> y/1
  Sum2/1 -> Sum/2, Delay/1
  Feedforward/1 -> Sum2/1

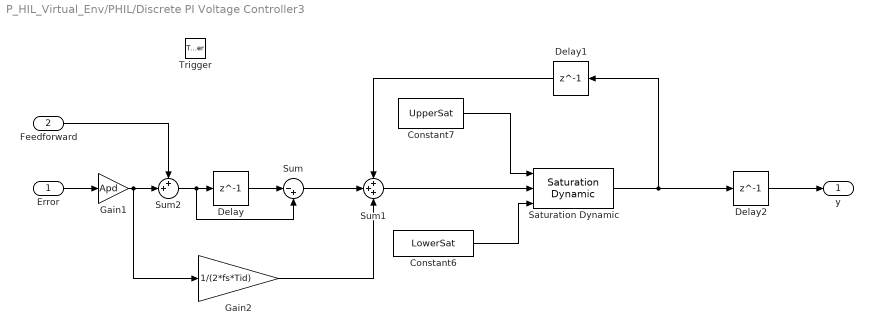
== system P_HIL_Virtual_Env/PHIL/Discrete PI Voltage Controller3 ==
  Error : Inport
  Feedforward : Inport  Port=2
  Trigger : TriggerPort  TriggerType=either  VariantControl=Variant  PortDimensions=1
  Constant6 : Constant  Value=LowerSat
  Constant7 : Constant  Value=UpperSat
  Delay : Delay  DelayLength=1
  Delay1 : Delay  DelayLength=1
  Delay2 : Delay  DelayLength=1
  Gain1 : Gain  Gain=Apd
  Gain2 : Gain  Gain=1/(2*fs*Tid)
  Saturation Dynamic : simulink/Discontinuities/Saturation Dynamic  OutMin=[]  OutMax=[]  OutDataTypeStr=Inherit: Same as second input  OutDataType=fixdt(1, 16)  OutScaling=2^-10  DoSatur=off
  Sum : Sum  Inputs=|-+
  Sum1 : Sum  Inputs=+++
  Sum2 : Sum  Inputs=++|
  y : Outport
  wires:
  Error/1 -> Gain1/1
  Gain1/1 -> Sum2/2, Gain2/1
  Sum1/1 -> Saturation Dynamic/2
  Saturation Dynamic/1 -> Delay1/1, Delay2/1
  Constant7/1 -> Saturation Dynamic/1
  Constant6/1 -> Saturation Dynamic/3
  Delay/1 -> Sum/1
  Sum/1 -> Sum1/2
  Gain2/1 -> Sum1/3
  Delay1/1 -> Sum1/1
  Delay2/1 -> y/1
  Sum2/1 -> Sum/2, Delay/1
  Feedforward/1 -> Sum2/1

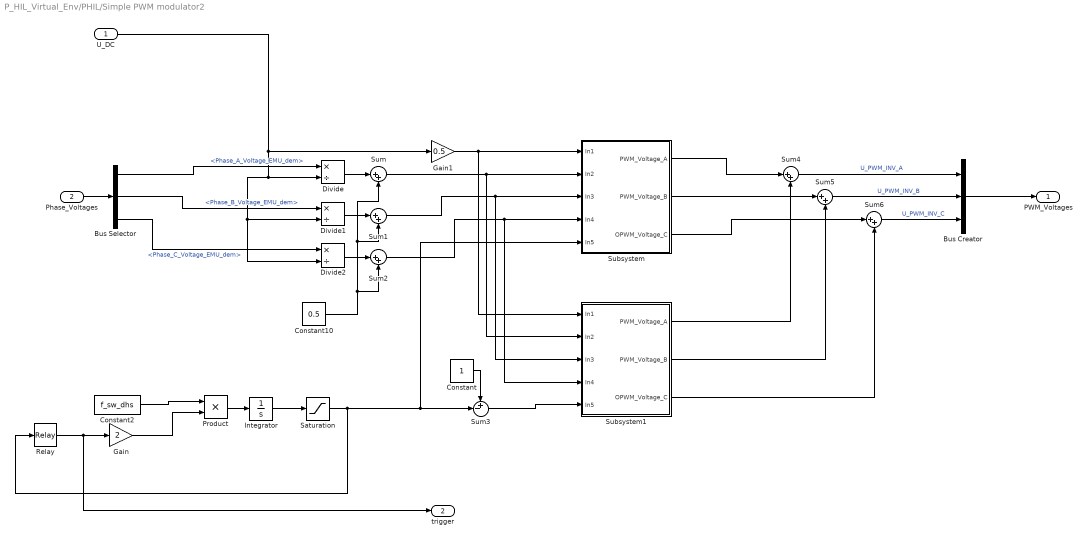
== system P_HIL_Virtual_Env/PHIL/Simple PWM modulator2 ==
  U_DC : Inport
  Phase_Voltages : Inport  Port=2
  Bus Creator : BusCreator  Inputs=3
  Bus Selector : BusSelector  OutputSignals=Phase_A_Voltage_EMU_dem,Phase_B_Voltage_EMU_dem,Phase_C_Voltage_EMU_dem
  Constant : Constant
  Constant10 : Constant  Value=0.5
  Constant2 : Constant  Value=f_sw_dhs
  Divide : Product  Inputs=*/
  Divide1 : Product  Inputs=*/
  Divide2 : Product  Inputs=*/
  Gain : Gain  Gain=2
  Gain1 : Gain  Gain=0.5
  Integrator : Integrator
  Product : Product
  Relay : Relay  OnSwitchValue=1  OffSwitchValue=0  OnOutputValue=-1  OffOutputValue=1
  Saturation : Saturate  UpperLimit=1  LowerLimit=0
  Subsystem : Subsystem
  Subsystem1 : Subsystem
  Sum{,1..2,4..6} (6 alike) : Sum  Inputs=|++
  Sum3 : Sum  Inputs=+-|
  PWM_Voltages : Outport
  trigger : Outport  Port=2
  wires:
  Constant2/1 -> Product/1
  Product/1 -> Integrator/1
  Integrator/1 -> Saturation/1
  Divide1/1 -> Sum1/1
  Saturation/1 -> Subsystem/5(In5), Sum3/2, Relay/1
  Relay/1 -> trigger/1, Gain/1
  Constant10/1 -> Sum2/2, Sum1/2, Sum/2
  Bus Selector/1 -> Divide/1  "<Phase_A_Voltage_EMU_dem>"
  Gain/1 -> Product/2
  Divide2/1 -> Sum2/1
  Divide/1 -> Sum/1
  Bus Selector/3 -> Divide2/1  "<Phase_C_Voltage_EMU_dem>"
  Bus Selector/2 -> Divide1/1  "<Phase_B_Voltage_EMU_dem>"
  Phase_Voltages/1 -> Bus Selector/1
  Bus Creator/1 -> PWM_Voltages/1
  Constant/1 -> Sum3/1
  Sum/1 -> Subsystem1/2(In2), Subsystem/2(In2)
  Sum1/1 -> Subsystem1/3(In3), Subsystem/3(In3)
  Sum2/1 -> Subsystem1/4(In4), Subsystem/4(In4)
  Sum3/1 -> Subsystem1/5(In5)
  Sum4/1 -> Bus Creator/1  "U_PWM_INV_A"
  Subsystem/1(PWM_Voltage_A) -> Sum4/1
  Subsystem1/1(PWM_Voltage_A) -> Sum4/2
  Sum5/1 -> Bus Creator/2  "U_PWM_INV_B"
  Subsystem/2(PWM_Voltage_B) -> Sum5/1
  Subsystem1/2(PWM_Voltage_B) -> Sum5/2
  Sum6/1 -> Bus Creator/3  "U_PWM_INV_C"
  Subsystem/3(OPWM_Voltage_C) -> Sum6/1
  Subsystem1/3(OPWM_Voltage_C) -> Sum6/2
  U_DC/1 -> Gain1/1, Divide2/2, Divide1/2, Divide/2
  Gain1/1 -> Subsystem1/1(In1), Subsystem/1(In1)

== system P_HIL_Virtual_Env/PHIL/3 phase LCL/L_C_L filter with current load ==
  U_INV : Inport
  U_DUT : Inport  Port=2
  Gain1 : Gain  Gain=1/L_dhs
  Gain3 : Gain  Gain=1/L_drom
  Gain4 : Gain  Gain=1/C_dhs
  Integrator : Integrator
  Integrator2 : Integrator
  Integrator3 : Integrator
  Subtract : Sum  Inputs=|+-
  Subtract2 : Sum  Inputs=|+-
  Subtract3 : Sum  Inputs=|++
  I_INV : Outport
  U_Phase : Outport  Port=2
  I_DUT : Outport  Port=3
  wires:
  Subtract/1 -> Gain1/1
  Gain1/1 -> Integrator/1
  Integrator/1 -> Subtract3/2, I_INV/1
  U_INV/1 -> Subtract/1
  U_DUT/1 -> Subtract2/1
  Subtract2/1 -> Gain3/1
  Gain3/1 -> Integrator2/1
  Integrator2/1 -> I_DUT/1, Subtract3/1
  Subtract3/1 -> Gain4/1
  Gain4/1 -> Integrator3/1
  Integrator3/1 -> Subtract2/2, Subtract/2, U_Phase/1

== system P_HIL_Virtual_Env/PHIL/3 phase LCL/L_C_L filter with current load1 ==
  U_INV : Inport
  U_DUT : Inport  Port=2
  Gain1 : Gain  Gain=1/L_dhs
  Gain3 : Gain  Gain=1/L_drom
  Gain4 : Gain  Gain=1/C_dhs
  Integrator : Integrator
  Integrator2 : Integrator
  Integrator3 : Integrator
  Subtract : Sum  Inputs=|+-
  Subtract2 : Sum  Inputs=|+-
  Subtract3 : Sum  Inputs=|++
  I_INV : Outport
  U_Phase : Outport  Port=2
  I_DUT : Outport  Port=3
  wires:
  Subtract/1 -> Gain1/1
  Gain1/1 -> Integrator/1
  Integrator/1 -> Subtract3/2, I_INV/1
  U_INV/1 -> Subtract/1
  U_DUT/1 -> Subtract2/1
  Subtract2/1 -> Gain3/1
  Gain3/1 -> Integrator2/1
  Integrator2/1 -> I_DUT/1, Subtract3/1
  Subtract3/1 -> Gain4/1
  Gain4/1 -> Integrator3/1
  Integrator3/1 -> Subtract2/2, Subtract/2, U_Phase/1

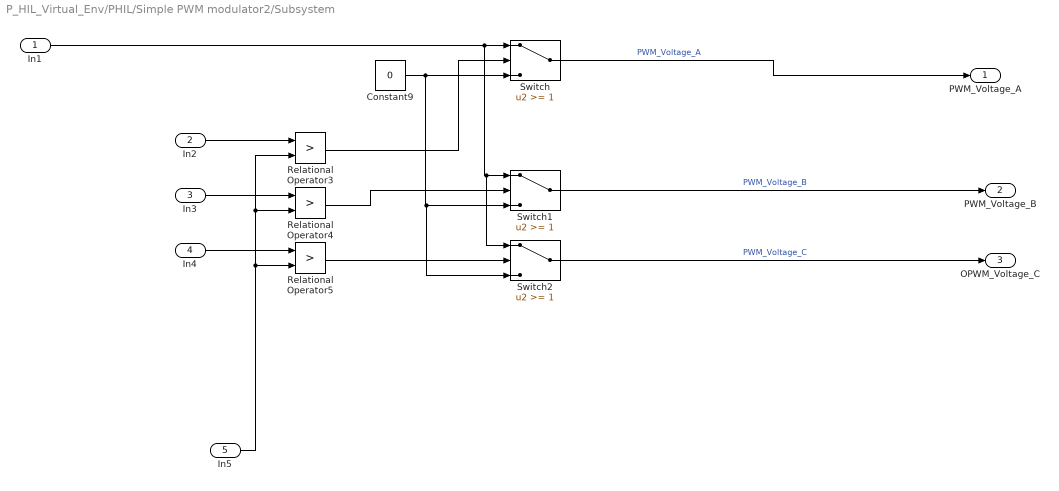
== system P_HIL_Virtual_Env/PHIL/Simple PWM modulator2/Subsystem ==
  In1 : Inport
  In2 : Inport  Port=2
  In3 : Inport  Port=3
  In4 : Inport  Port=4
  In5 : Inport  Port=5
  Constant9 : Constant  Value=0
  Relational Operator3 : RelationalOperator  Operator=>  OutDataTypeStr=boolean  RndMeth=Simplest
  Relational Operator4 : RelationalOperator  Operator=>  OutDataTypeStr=boolean  RndMeth=Simplest
  Relational Operator5 : RelationalOperator  Operator=>  OutDataTypeStr=boolean  RndMeth=Simplest
  Switch : Switch  Threshold=1
  Switch1 : Switch  Threshold=1
  Switch2 : Switch  Threshold=1
  PWM_Voltage_A : Outport
  PWM_Voltage_B : Outport  Port=2
  OPWM_Voltage_C : Outport  Port=3
  wires:
  Relational Operator4/1 -> Switch1/2
  In5/1 -> Relational Operator3/2, Relational Operator4/2, Relational Operator5/2
  Constant9/1 -> Switch2/3, Switch1/3, Switch/3
  Relational Operator3/1 -> Switch/2
  In3/1 -> Relational Operator4/1
  Relational Operator5/1 -> Switch2/2
  Switch/1 -> PWM_Voltage_A/1  "PWM_Voltage_A"
  In1/1 -> Switch2/1, Switch1/1, Switch/1
  In2/1 -> Relational Operator3/1
  In4/1 -> Relational Operator5/1
  Switch1/1 -> PWM_Voltage_B/1  "PWM_Voltage_B"
  Switch2/1 -> OPWM_Voltage_C/1  "PWM_Voltage_C"

== system P_HIL_Virtual_Env/PHIL/Simple PWM modulator2/Subsystem1 ==
  In1 : Inport
  In2 : Inport  Port=2
  In3 : Inport  Port=3
  In4 : Inport  Port=4
  In5 : Inport  Port=5
  Constant9 : Constant  Value=0
  Relational Operator3 : RelationalOperator  Operator=>  OutDataTypeStr=boolean  RndMeth=Simplest
  Relational Operator4 : RelationalOperator  Operator=>  OutDataTypeStr=boolean  RndMeth=Simplest
  Relational Operator5 : RelationalOperator  Operator=>  OutDataTypeStr=boolean  RndMeth=Simplest
  Switch : Switch  Threshold=1
  Switch1 : Switch  Threshold=1
  Switch2 : Switch  Threshold=1
  PWM_Voltage_A : Outport
  PWM_Voltage_B : Outport  Port=2
  OPWM_Voltage_C : Outport  Port=3
  wires:
  Relational Operator4/1 -> Switch1/2
  In5/1 -> Relational Operator3/2, Relational Operator4/2, Relational Operator5/2
  Constant9/1 -> Switch2/3, Switch1/3, Switch/3
  Relational Operator3/1 -> Switch/2
  In3/1 -> Relational Operator4/1
  Relational Operator5/1 -> Switch2/2
  Switch/1 -> PWM_Voltage_A/1  "PWM_Voltage_A"
  In1/1 -> Switch2/1, Switch1/1, Switch/1
  In2/1 -> Relational Operator3/1
  In4/1 -> Relational Operator5/1
  Switch1/1 -> PWM_Voltage_B/1  "PWM_Voltage_B"
  Switch2/1 -> OPWM_Voltage_C/1  "PWM_Voltage_C"
